simulink model "Cyber_Physical_Microgrid"  (R2024b)
settings: Solver=VariableStepAuto  StartTime=0.0  StopTime=270  RelTol=1e-3
values from neighbouring files (symbols this model uses):
  Bat =     [initData.mat]
  droopFC1 = 0.05    [initData.mat]
  droopFC2 = 0.05    [initData.mat]
  droopP2 = 0.05    [initData.mat]
  droopQ1 = 0.05    [initData.mat]
  droopQ2 = 0.05    [initData.mat]
  Pref2 = 0.8    [initData.mat]
  Qref1 = 0    [initData.mat]
  Qref2 = 0    [initData.mat]
  timeACLoadCurtail = 200    [initData.mat]
  timeSolarCurtail = 200    [initData.mat]
  Ts = 5e-05    [initData.mat]
  Ts_AC = 0.0002    [initData.mat]
  Ts_DC = 0.001    [initData.mat]
  volt2 = [270.467186401 250.166401688 246.278575679 243.847178474 242.073246789 240.654489675 239.457734124 238.414696845 237.485238449 236.643553985 235.871256975 235.151075236 ... (161 elements, 1x161)]    [initData.mat]
undefined symbols (not defined in the file or in its folder): BattTempBp, CapLUTBp, CapSOCBp, DiscIntNeverNeededParam, Em, Np, Ns, RInt, Tc_Batt
libraries: nesl_utility x55, fl_lib x52, ee_lib x39, modbuslib x16, spsRMSLib x8, simulink x5, spsFourierLib x2, batteryecm_lib x1, eeTransforms x1
(part 1 of 3)
settings Model: Creator=dines  LastModifiedBy=dines
settings ConfigSetCC: ModbusTableInfo=[]

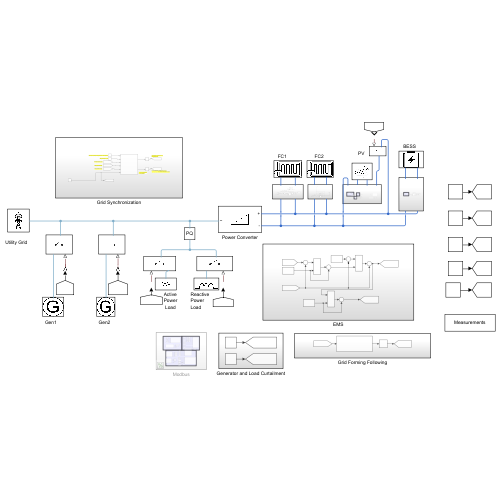
[thumbnail: Simulink's stored preview of the top-level diagram]
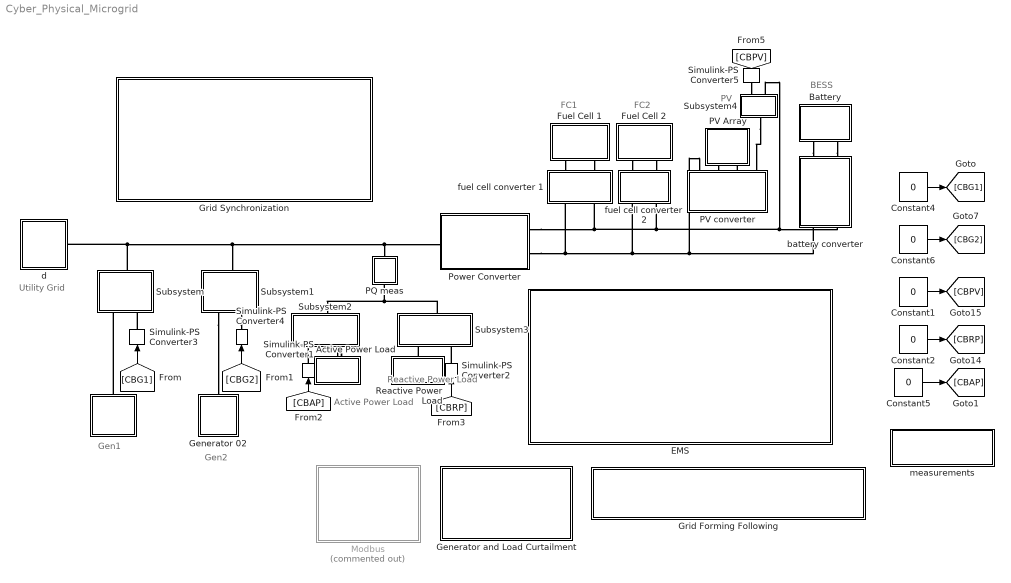
== system Cyber_Physical_Microgrid ==
  note: Gen1
  note: BESS
  note: PV
  note: FC1
  note: Reactive
      | Power
      | Load
  note: Gen2
  note: Active
      | Power
      |  Load
  note: FC2
  note: Utility Grid
  " " : Subsystem
      mask Display: image('generator.jpeg');
  Active Power Load : Subsystem
      mask Display: image('Resistor_symbol_America.svg.png');
  Battery : Subsystem
      mask Display: image('46518.png');
  Constant{1..2,4..6} (5 alike) : Constant  Value=0
  EMS : Subsystem
  Fuel Cell 1 : Subsystem
      mask Display: image('6255645.png');
  Fuel Cell 2 : Subsystem
      mask Display: image('6255645.png');
  Generator 02 : Subsystem
      mask Display: image('generator.jpeg');
  Generator and Load Curtailment : Subsystem
  Grid Forming Following : Subsystem
  Grid Synchronization : Subsystem
  Modbus : Subsystem  Commented=on
  PQ meas : Subsystem
      mask Display: disp('PQ')
  PV Array : Subsystem
      mask Display: image('solar-panel-icon-design-renewable-energy-sign-and-symbol-vector.jpg');
  PV converter : Subsystem
  Power Converter : Subsystem
      mask Display: image('743.s.png');
  Reactive Power Load : Subsystem
      mask Display: image('Inductor_symbol.svg.png');
  Simulink-PS Converter{1..5} (5 alike) : nesl_utility/Simulink-PS Converter  PhysicalDomain=network_engine_domain  SubClassName=ps_input  LeftPortType=input  RightPortType=output  PseudoPeriodic=off  Frequencies=[]  NoiseDistribution=none  NoiseParameters=[]  Unit=1  AffineConversion=off  FilteringAndDerivatives=provide  SimscapeFilterOrder=1  InputFilterTimeConstant=0.001  UdotUserProvided=0
  Subsystem : Subsystem
      mask Display: image('p0dz3vs9.png');
  Subsystem1 : Subsystem
      mask Display: image('p0dz3vs9.png');
  Subsystem2 : Subsystem
      mask Display: image('p0dz3vs9.png');
  Subsystem3 : Subsystem
      mask Display: image('p0dz3vs9.png');
  Subsystem4 : Subsystem
      mask Display: image('p0dz3vs9.png');
  battery converter : Subsystem
  d : Subsystem
      mask Display: image('utility.jpg');
  fuel cell converter 1 : Subsystem
  fuel cell converter 2 : Subsystem
  measurements : Subsystem
      mask Display: disp('Measurements')
  wires:
  [CBG2] -> Simulink-PS Converter4/1
  [CBG1] -> Simulink-PS Converter3/1
  Constant6/1 -> [CBG2]
  [CBAP] -> Simulink-PS Converter1/1
  Constant2/1 -> [CBRP]
  Constant1/1 -> [CBPV]
  [CBRP] -> Simulink-PS Converter2/1
  Constant4/1 -> [CBG1]
  Constant5/1 -> [CBAP]
  connections:
  fuel cell converter 2/RConn2 -- Subsystem4/LConn2 -- battery converter/RConn2 -- fuel cell converter 1/RConn2 -- Power Converter/RConn1
  PQ meas/LConn1 -- Power Converter/LConn1 -- Subsystem/RConn1 -- d/RConn1 -- Subsystem1/RConn1
  PV converter/LConn1 -- Power Converter/RConn2 -- fuel cell converter 1/RConn1 -- fuel cell converter 2/RConn1 -- battery converter/RConn1
  PQ meas/RConn1 -- Subsystem2/RConn1 -- Subsystem3/RConn1
  Battery/RConn2 -- battery converter/LConn2
  Simulink-PS Converter5/RConn1 -- Subsystem4/LConn1
  Simulink-PS Converter3/RConn1 -- Subsystem/LConn2
  Simulink-PS Converter1/RConn1 -- Subsystem2/LConn1
  PV converter/LConn3 -- PV Array/LConn2
  PV Array/LConn1 -- PV converter/LConn2
  Reactive Power Load/LConn1 -- Subsystem3/LConn1
  " "/RConn1 -- Subsystem/LConn1
  Subsystem2/LConn2 -- Active Power Load/LConn1
  Subsystem1/LConn2 -- Simulink-PS Converter4/RConn1
  Fuel Cell 1/RConn2 -- fuel cell converter 1/LConn2
  Battery/RConn1 -- battery converter/LConn1
  Fuel Cell 1/RConn1 -- fuel cell converter 1/LConn1
  Fuel Cell 2/RConn1 -- fuel cell converter 2/LConn1
  Fuel Cell 2/RConn2 -- fuel cell converter 2/LConn2
  Simulink-PS Converter2/RConn1 -- Subsystem3/LConn2
  Subsystem1/LConn1 -- Generator 02/RConn1
  Subsystem4/RConn1 -- PV converter/LConn4

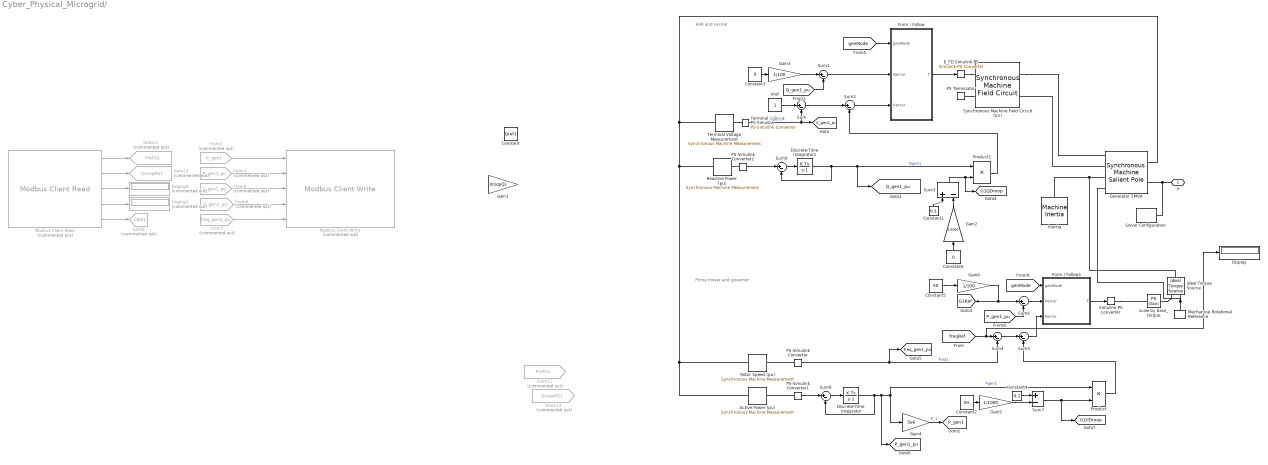
== system Cyber_Physical_Microgrid/  ==
  note: Prime mover
      | and governor
  note: AVR and exciter
  "Active Power (pu) " : ee_lib/Electromechanical/Synchronous/Synchronous Machine Measurement  output_idx=12
      settings: InternalSimscapePortConfiguration="{\"Bottom\":[],\"Left\":[{\"id\":\"pu_input\",\"label\":\"pu\",\"type\":\"input\"}],\"Right\":[{\"id\":\"pu_output\",\"label\":\"o\",\"type\":\"output\"}],\"Top\":[]}"
  Constant : Constant  Value=Qref1
  Constant1 : Constant  Value=0.1
  Constant2 : Constant  Value=50
  Constant3 : Constant  Value=0
  Constant4 : Constant  Value=0.1
  Constant5 : Constant  Value=50
  Constant6 : Constant  Value=0
  Discrete-Time Integrator : DiscreteIntegrator  gainval=20  SampleTime=Ts_AC  ICPrevOutput=DiscIntNeverNeededParam  ICPrevScaledInput=DiscIntNeverNeededParam
  Discrete-Time Integrator1 : DiscreteIntegrator  gainval=20  SampleTime=Ts_AC  ICPrevOutput=DiscIntNeverNeededParam  ICPrevScaledInput=DiscIntNeverNeededParam
  Display : Display
  Display2 : Display  Commented=on
      settings: Format=decimal (Stored Integer)  Decimation=4
  Display6 : Display  Commented=on
      settings: Format=decimal (Stored Integer)  Decimation=4
  "E_FD Simulink-PS " : nesl_utility/Simulink-PS Converter  PhysicalDomain=network_engine_domain  SubClassName=ps_input  LeftPortType=input  RightPortType=output  PseudoPeriodic=off  Frequencies=[]  NoiseDistribution=none  NoiseParameters=[]  Unit=1  AffineConversion=off  FilteringAndDerivatives=provide  SimscapeFilterOrder=1  InputFilterTimeConstant=.001  UdotUserProvided=0
  Form / Follow : Subsystem
  Form / Follow1 : Subsystem
  From11 : From  Commented=on  GotoTag=PrefG1
  From12 : From  Commented=on  GotoTag=DroopPG1
  From2 : From  Commented=on  GotoTag=P_gen1  TagVisibility=global
  From3 : From  Commented=on  GotoTag=P_gen1_pu  TagVisibility=global
  From4 : From  Commented=on  GotoTag=V_gen1_pu  TagVisibility=global
  From6 : From  Commented=on  GotoTag=Q_gen1_pu  TagVisibility=global
  From7 : From  Commented=on  GotoTag=freq_gen1_pu  TagVisibility=global
  Gain1 : Gain  Gain=droopQ1
  Gain2 : Gain  Gain=1/1000
  Gain3 : Gain  Gain=1/100
  Gain4 : Gain  Gain=5e6
  Gain5 : Gain  Gain=1/1000
  Gain6 : Gain  Gain=1/100
  Generator 5MVA : ee_lib/Electromechanical/Synchronous/Synchronous Machine Salient Pole  port_option=ee.enum.threePhasePort.composite  SRated=5e6 A*V  VRated=6600 V  FRated=50 Hz  nPolePairs=4  param_option=ee.enum.sm.parameterization.standard  fieldCircuitParameterization_option=ee.enum.sm.fieldparameterization.current  baseEfd=216.54 V  baseIfd=50 A  zero_sequence=ee.enum.park.zerosequence.exclude  axes_param=ee.enum.rotorangle.daxis  Ladu=0.9  Laqu=0.55  L0=0.15  Ll=0.15  Ra=0.011  Lfd=0.2571  Rfd=0.0006  L1d=0.2  R1d=0.0354  L1q=0.2567  R1q=0.0428  Xl=0.15  Xd=1.05  Xq=0.7  X0=0.15  Xdd=0.35  Xddd=0.25  Xqdd=0.325  d_option=ee.enum.circuit.open  Td0d=5.25 s  Tdd=1.75 s  Td0dd=0.03 s  Tddd=0.0214 s  q_option=ee.enum.circuit.open  Tq0dd=0.05 s  Tqdd=0.0232 s  saturation_option=ee.enum.saturation.exclude  saturation_ifd=[0.00, 0.48, 0.76, 1.38, 1.79]  saturation_Vag=[0.00, 0.43, 0.59, 0.71, 0.76]  initialization_option=ee.enum.sm.initialization.electrical  source_type=ee.enum.sm.load_flow_source_type.Swing  Vmag0=6600 V  Vang0=0 deg  Pt0=0.5 A*V  Qt0=0 A*V  minimum_pu=0.95  phase_search_range=[-inf, inf] deg  gmin=1e-6 S  connection_option=ee.enum.Connection.wye  num_q_dampers=1  rotor_offset=-pi / 2 rad  pu_psid_specify=on  pu_psid_priority=High  pu_psid=0  pu_psid_nominal_specify=off  pu_psid_nominal_value=1  pu_psid_nominal_unit=1  pu_psiq_specify=on  pu_psiq_priority=High  pu_psiq=0  pu_psiq_nominal_specify=off  pu_psiq_nominal_value=1  pu_psiq_nominal_unit=1  pu_psifd_specify=on  pu_psifd_priority=High  pu_psifd=0  pu_psifd_nominal_specify=off  pu_psifd_nominal_value=1  pu_psifd_nominal_unit=1  pu_psi1d_specify=on  pu_psi1d_priority=High  pu_psi1d=0  pu_psi1d_nominal_specify=off  pu_psi1d_nominal_value=1  pu_psi1d_nominal_unit=1  pu_psi1q_specify=on  pu_psi1q_priority=High  pu_psi1q=0  pu_psi1q_nominal_specify=off  pu_psi1q_nominal_value=1  pu_psi1q_nominal_unit=1  angular_position_diff_specify=on  angular_position_diff_priority=High  angular_position_diff=0 deg  angular_position_diff_nominal_specify=off  angular_position_diff_nominal_value=1  angular_position_diff_nominal_unit=deg  Tmeas=298.15 K  alpha=3.93e-3 1/K  stator_thermal_mass=100 J/K  rotor_thermal_mass=200 J/K  temperatureA_specify=off  temperatureA_priority=High  temperatureA=25 degC  temperatureA_nominal_specify=off  temperatureA_nominal_value=1  temperatureA_nominal_unit=degC  temperatureB_specify=off  temperatureB_priority=High  temperatureB=25 degC  temperatureB_nominal_specify=off  temperatureB_nominal_value=1  temperatureB_nominal_unit=degC  temperatureC_specify=off  temperatureC_priority=High  temperatureC=25 degC  temperatureC_nominal_specify=off  temperatureC_nominal_value=1  temperatureC_nominal_unit=degC  temperatureR_specify=off  temperatureR_priority=High  temperatureR=25 degC  temperatureR_nominal_specify=off  temperatureR_nominal_value=1  temperatureR_nominal_unit=degC
      settings: LogSimulationData=on  InternalSimscapePortConfiguration="{\"Bottom\":[],\"Left\":[{\"id\":\"fd_p\",\"label\":\"fd+\",\"type\":\"foundation.electrical.electrical\"},{\"id\":\"fd_n\",\"label\":\"fd-\",\"type\":\"foundation.electrical.electrical\"},{\"id\":\"R\",\"label\":\"R\",\"type\":\"foundation.mechanical.rotational.rotational\"},{\"id\":\"C\",\"label\":\"C\",\"type\":\"foundation.mechanical.rotational.rotational\"}],\"Right\":[{\"id\":\"pu_output\",\"label\":\"pu\",\"type\":\"output\"},{\"id\":\"N\",\"label\":\"~\",\"type\":\"foundation.electrical.three_phase\"}],\"Top\":[]}"
  Goto12 : Goto  Commented=on  GotoTag=PrefG1  TagVisibility=global
  Goto13 : Goto  Commented=on  GotoTag=DroopPG1  TagVisibility=global
  Goto8 : Goto  Commented=on  GotoTag=CBG1  TagVisibility=global
  Ideal Torque Source : fl_lib/Mechanical/Mechanical Sources/Ideal Torque Source
  Inertia : ee_lib/Electromechanical/Mechanical/Machine Inertia  SRated=5e6 V*A  FRated=50 Hz  nPolePairs=4  inertia_option=2  J=27548 kg*m^2  H=3.525 s*W/V/A  damper_option=2  D=39.0509 N*m/(rad/s)  pu_D=0.01  initialization_option=2  fMechanical0=50 Hz  fElectrical0=50 Hz
      settings: LogSimulationData=on  InternalSimscapePortConfiguration="{\"Bottom\":[],\"Left\":[{\"id\":\"R\",\"label\":\"R\",\"type\":\"foundation.mechanical.rotational.rotational\"}],\"Right\":[],\"Top\":[]}"
  Mechanical Rotational Reference : fl_lib/Mechanical/Rotational Elements/Mechanical Rotational Reference
  Modbus Client Read : modbuslib/Modbus Client Read  Commented=on  RetainClient=No Modbus client available  ClientList=No Modbus client available  ConnectionEndpoint=No Modbus client selected  ServerId=1  RegisterTable={ '1', 'PrefG1', '21', 'Holding Register', 'double', '1'; '2', 'DroopPG1', '25', 'Holding Register', 'double', '1'; '3', 'QrefG1', '29', 'Holding Register', 'double', '1'; '4', 'DroopQG1', '34', 'Holding Register', 'double', '1'; '5', 'CBG1', '38', 'Coil', 'bit', '1' }  SampleTime=1
  Modbus Client Write : modbuslib/Modbus Client Write  Commented=on  RetainClient=No Modbus client available  ClientList=No Modbus client available  ConnectionEndpoint=No Modbus client selected  ServerId=1  RegisterTable={ '1', 'P_gen1', '1', 'Holding Register', 'double'; '2', 'P_gen1_pu', '5', 'Holding Register', 'double'; '3', 'V_gen1_pu', '9', 'Holding Register', 'double'; '4', 'Q_gen1_pu', '13', 'Holding Register', 'double'; '5', 'freq_gen1_pu', '17', 'Holding Register', 'double' }  SampleTime=1
  PS Terminator : fl_lib/Physical Signals/Sinks/PS Terminator
  PS-Simulink Converter : nesl_utility/PS-Simulink Converter  PhysicalDomain=network_engine_domain  SubClassName=ps_output  LeftPortType=input  RightPortType=output  PseudoPeriodic=off  Frequencies=[]  VectorFormat=1-D array  Unit=inherit  AffineConversion=off
  PS-Simulink Converter1 : nesl_utility/PS-Simulink Converter  PhysicalDomain=network_engine_domain  SubClassName=ps_output  LeftPortType=input  RightPortType=output  PseudoPeriodic=off  Frequencies=[]  VectorFormat=1-D array  Unit=inherit  AffineConversion=off
  PS-Simulink Converter2 : nesl_utility/PS-Simulink Converter  PhysicalDomain=network_engine_domain  SubClassName=ps_output  LeftPortType=input  RightPortType=output  PseudoPeriodic=off  Frequencies=[]  VectorFormat=1-D array  Unit=inherit  AffineConversion=off
  Product : Product
  Product1 : Product
  Reactive Power (pu) : ee_lib/Electromechanical/Synchronous/Synchronous Machine Measurement  output_idx=13
      settings: InternalSimscapePortConfiguration="{\"Bottom\":[],\"Left\":[{\"id\":\"pu_input\",\"label\":\"pu\",\"type\":\"input\"}],\"Right\":[{\"id\":\"pu_output\",\"label\":\"o\",\"type\":\"output\"}],\"Top\":[]}"
  Rotor Speed (pu) : ee_lib/Electromechanical/Synchronous/Synchronous Machine Measurement  output_idx=4
      settings: InternalSimscapePortConfiguration="{\"Bottom\":[],\"Left\":[{\"id\":\"pu_input\",\"label\":\"pu\",\"type\":\"input\"}],\"Right\":[{\"id\":\"pu_output\",\"label\":\"o\",\"type\":\"output\"}],\"Top\":[]}"
  Simulink-PS Converter : nesl_utility/Simulink-PS Converter  PhysicalDomain=network_engine_domain  SubClassName=ps_input  LeftPortType=input  RightPortType=output  PseudoPeriodic=off  Frequencies=[]  NoiseDistribution=none  NoiseParameters=[]  Unit=1  AffineConversion=off  FilteringAndDerivatives=provide  SimscapeFilterOrder=1  InputFilterTimeConstant=0.001  UdotUserProvided=0
  Solver Configuration : nesl_utility/Solver Configuration  PhysicalDomain=network_engine_domain  SubClassName=solver  LeftPortType=input  RightPortType=generic  Tones=[]  Harmonics=[]  SimulateNoise=off  Profile=off  UseLocalSampling=off  EnableSwitchedLinearOptims=on  FrequencyDomain=off  UseCCode=off  RelTol=0.001  AbsTol=1e-06  MinStep=1e-09  ToWorkspace=off  RevertToSquareIcSolve=off  NumHomotopyIterations=100  PhasorMode=off  PhasorModeNumHarmonics=1  ConsistencySolver=NEWTON_FTOL  IndexReductionMethod=DerivativeReplacement  DoDC=off  ResidualTolerance=1e-09  ConsistencyTolSource=GLOBAL  ConsistencyAbsTol=0.001  ConsistencyRelTol=0.001  ConsistencyTolFactor=0.001  UseLocalSolver=on  LocalSolverChoice=NE_PARTITIONING_ADVANCER  ResolveIndetEquations=on  FunctionEvalNumThread=1  LocalSolverSampleTime=Ts_DC  DoFixedCost=on  MaxNonlinIter=1  MaxModeIter=2  ComputeImpulses=off  ImpulseIterations=2  LinearAlgebra=auto  LinearAlgebraNumThread=0  EquationFormulation=NE_TIME_EF  DelaysMemoryBudget=1024  AutomaticFiltering=on  FilteringTimeConstant=0.001  PartitionStorageMethod=AS_NEEDED  PartitionMemoryBudget=1024  PartitionMethod=ROBUST  MultibodyUseLocalSolver=off  MultibodyLocalSolverChoice=ODE1  MultibodyLocalSolverSampleTime=0.001
  Sum{,1..2,4..6,8..9} (8 alike) : Sum  Inputs=|+-
  Sum3 : Sum  Inputs=+-
  Sum7 : Sum  Inputs=+-
  Synchronous Machine Field Circuit (pu) : ee_lib/Electromechanical/Synchronous/Synchronous Machine Field Circuit  unit_option=ee.enum.unit.pu  SRated=5e6 V*A  FRated=50 Hz  fieldCircuitParameterization_option=2  baseEfd=92.95 V  baseIfd=50 A  parameterization_option=2  Ladu=1.66  Rfd=0.0006  Xl=0.15  Xd=1.05  Xdd=0.35  Xddd=0.23  d_option=ee.enum.circuit.open  Td0d=5.25 s  Tdd=1.3260 s  Td0dd=0.03 s  Tddd=0.0230 s
      settings: LogSimulationData=on  InternalSimscapePortConfiguration="{\"Bottom\":[],\"Left\":[{\"id\":\"Efd_pu\",\"label\":\"Efd_pu\",\"type\":\"input\"},{\"id\":\"Ifd_pu\",\"label\":\"Ifd_pu\",\"type\":\"output\"}],\"Right\":[{\"id\":\"fd_p\",\"label\":\"fd+\",\"type\":\"foundation.electrical.electrical\"},{\"id\":\"fd_n\",\"label\":\"fd-\",\"type\":\"foundation.electrical.electrical\"}],\"Top\":[]}"
  Terminal Voltage Measurement : ee_lib/Electromechanical/Synchronous/Synchronous Machine Measurement  output_idx=14
      settings: LogSimulationData=on  InternalSimscapePortConfiguration="{\"Bottom\":[],\"Left\":[{\"id\":\"pu_input\",\"label\":\"pu\",\"type\":\"input\"}],\"Right\":[{\"id\":\"pu_output\",\"label\":\"o\",\"type\":\"output\"}],\"Top\":[]}"
  Terminal Voltage PS-Simulink : nesl_utility/PS-Simulink Converter  PhysicalDomain=network_engine_domain  SubClassName=ps_output  LeftPortType=input  RightPortType=output  PseudoPeriodic=off  Frequencies=[]  VectorFormat=1-D array  Unit=1  AffineConversion=off
  Vref : Constant  SampleTime=Ts_AC
  scale by base_torque : fl_lib/Physical Signals/Functions/PS Gain  gain=63661.97724 N*m
  a : PMIOPort  Side=Right
  tag scope: G1PDroop=global, G1QDroop=global, G1Ref=global, P_gen1=global, P_gen1_pu=global, Q_gen1_pu=global, V_gen1_pu=global, freq_gen1_pu=global
  wires:
  Product1/1 -> Sum2/2
  Gain3/1 -> Sum1/1
  Gain2/1 -> Sum3/2
  Sum3/1 -> [G1QDroop], Product1/2
  Constant1/1 -> Sum3/1
  Constant6/1 -> Gain2/1
  Form / Follow/1(T) -> "E_FD Simulink-PS "/1
  [Q_gen1_pu] -> Sum1/2
  [genMode] -> Form / Follow/1(genMode)
  Sum1/1 -> Form / Follow/2(Qerror)
  Discrete-Time Integrator1/1 -> Product1/1, [Q_gen1_pu], Sum9/2  "Qgen1"
  Terminal Voltage PS-Simulink/1 -> [V_gen1_pu], Sum/2  "Vgen1"
  Sum2/1 -> Form / Follow/3(Verror)
  Sum/1 -> Sum2/1
  Vref/1 -> Sum/1
  Modbus Client Read/1 -> Goto12/1
  From7/1 -> Modbus Client Write/5
  From6/1 -> Modbus Client Write/4
  From4/1 -> Modbus Client Write/3
  From3/1 -> Modbus Client Write/2
  From2/1 -> Modbus Client Write/1
  Gain6/1 -> Sum6/1, [G1Ref]
  Sum7/1 -> [G1PDroop], Product/2
  Gain5/1 -> Sum7/2
  Constant4/1 -> Sum7/1
  Form / Follow1/1(T) -> Simulink-PS Converter/1
  [genMode] -> Form / Follow1/1(genMode)
  Sum6/1 -> Form / Follow1/2(Perror)
  Sum5/1 -> Form / Follow1/3(Ferror)
  [P_gen1_pu] -> Sum6/2
  Gain4/1 -> [P_gen1]  "P_1"
  Discrete-Time Integrator/1 -> Gain4/1, Product/1, [P_gen1_pu], Sum8/2  "Pgen1"
  Product/1 -> Sum5/2
  Sum4/1 -> Sum5/1
  [freqRef] -> Display/1, Sum4/1
  PS-Simulink Converter/1 -> [freq_gen1_pu], Sum4/2  "freq1"
  Modbus Client Read/2 -> Goto13/1
  Modbus Client Read/5 -> Goto8/1
  Modbus Client Read/3 -> Display6/1
  Modbus Client Read/4 -> Display2/1
  Constant2/1 -> Gain5/1
  Constant5/1 -> Gain6/1
  PS-Simulink Converter1/1 -> Sum8/1
  Sum8/1 -> Discrete-Time Integrator/1
  Constant3/1 -> Gain3/1
  PS-Simulink Converter2/1 -> Sum9/1
  Sum9/1 -> Discrete-Time Integrator1/1
  connections:
  Synchronous Machine Field Circuit (pu)/RConn1 -- Generator 5MVA/LConn1
  Ideal Torque Source/LConn1 -- Generator 5MVA/LConn3 -- Inertia/LConn1
  Mechanical Rotational Reference/LConn1 -- Ideal Torque Source/RConn2 -- Generator 5MVA/LConn4
  Solver Configuration/RConn1 -- a/RConn1 -- Generator 5MVA/RConn2
  PS-Simulink Converter2/LConn1 -- Reactive Power (pu)/RConn1
  Terminal Voltage Measurement/RConn1 -- Terminal Voltage PS-Simulink/LConn1
  Rotor Speed (pu)/LConn1 -- "Active Power (pu) "/LConn1 -- Generator 5MVA/RConn1 -- Terminal Voltage Measurement/LConn1 -- Reactive Power (pu)/LConn1
  "E_FD Simulink-PS "/RConn1 -- Synchronous Machine Field Circuit (pu)/LConn1
  PS Terminator/LConn1 -- Synchronous Machine Field Circuit (pu)/LConn2
  Generator 5MVA/LConn2 -- Synchronous Machine Field Circuit (pu)/RConn2
  PS-Simulink Converter1/LConn1 -- "Active Power (pu) "/RConn1
  PS-Simulink Converter/LConn1 -- Rotor Speed (pu)/RConn1
  scale by base_torque/RConn1 -- Ideal Torque Source/RConn1
  Simulink-PS Converter/RConn1 -- scale by base_torque/LConn1

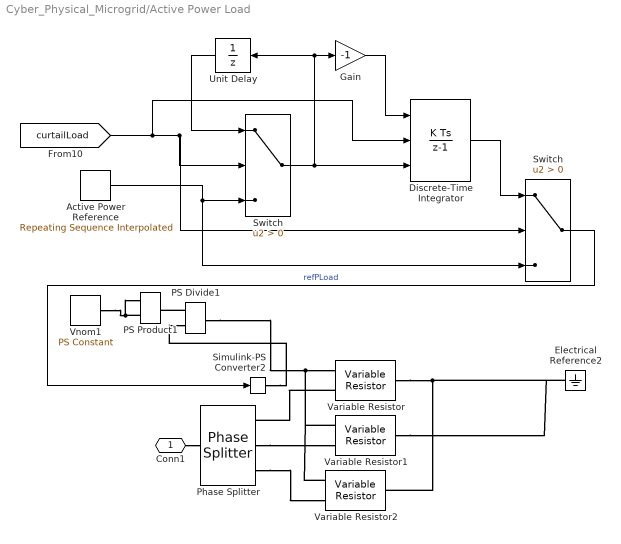
== system Cyber_Physical_Microgrid/Active Power Load ==
  Active Power Reference : simulink/Sources/Repeating Sequence Interpolated  OutValues=[1 1 10e6 10e6]  TimeValues=[0 1 5 500]  LookUpMeth=Interpolation-Use End Values  tsamp=Ts_AC  OutMin=[]  OutMax=[]  OutDataTypeStr=double  OutputDataTypeScalingMode=double  OutDataType=fixdt(0,8)  OutScaling=2^-10
  Discrete-Time Integrator : DiscreteIntegrator  gainval=1e-2  ExternalReset=rising  InitialConditionSource=external  SampleTime=-1  LimitOutput=on  LowerSaturationLimit=6e6  ICPrevOutput=DiscIntNeverNeededParam  ICPrevScaledInput=DiscIntNeverNeededParam
  Electrical Reference2 : fl_lib/Electrical/Electrical Elements/Electrical Reference
  Gain : Gain  Gain=-1
  PS Divide1 : fl_lib/Physical Signals/Functions/PS Divide
  PS Product1 : fl_lib/Physical Signals/Functions/PS Product
  Phase Splitter : ee_lib/Connectors & References/Phase Splitter
  Simulink-PS Converter2 : nesl_utility/Simulink-PS Converter  PhysicalDomain=network_engine_domain  SubClassName=ps_input  LeftPortType=input  RightPortType=output  PseudoPeriodic=off  Frequencies=[]  NoiseDistribution=none  NoiseParameters=[]  Unit=W  AffineConversion=off  FilteringAndDerivatives=provide  SimscapeFilterOrder=1  InputFilterTimeConstant=0.001  UdotUserProvided=0
  Switch : Switch  Criteria=u2 > Threshold  SaturateOnIntegerOverflow=off  InputSameDT=off
  "Switch " : Switch  Criteria=u2 > Threshold  SaturateOnIntegerOverflow=off  InputSameDT=off
  Unit Delay : UnitDelay  SampleTime=-1  HasFrameUpgradeWarning=on
  Variable Resistor : fl_lib/Electrical/Electrical Elements/Variable Resistor  Rmin=0 Ohm  thermalEnable=false  thermal_mass=1 J/K  i_specify=off  i_priority=None  i=0 A  i_nominal_specify=off  i_nominal_value=1  i_nominal_unit=A  v_specify=off  v_priority=None  v=0 V  v_nominal_specify=off  v_nominal_value=1  v_nominal_unit=V  T_specify=off  T_priority=None  T=300 K  T_nominal_specify=off  T_nominal_value=1  T_nominal_unit=K
  Variable Resistor1 : fl_lib/Electrical/Electrical Elements/Variable Resistor  Rmin=0 Ohm  thermalEnable=false  thermal_mass=1 J/K  i_specify=off  i_priority=None  i=0 A  i_nominal_specify=off  i_nominal_value=1  i_nominal_unit=A  v_specify=off  v_priority=None  v=0 V  v_nominal_specify=off  v_nominal_value=1  v_nominal_unit=V  T_specify=off  T_priority=None  T=300 K  T_nominal_specify=off  T_nominal_value=1  T_nominal_unit=K
  Variable Resistor2 : fl_lib/Electrical/Electrical Elements/Variable Resistor  Rmin=0 Ohm  thermalEnable=false  thermal_mass=1 J/K  i_specify=off  i_priority=None  i=0 A  i_nominal_specify=off  i_nominal_value=1  i_nominal_unit=A  v_specify=off  v_priority=None  v=0 V  v_nominal_specify=off  v_nominal_value=1  v_nominal_unit=V  T_specify=off  T_priority=None  T=300 K  T_nominal_specify=off  T_nominal_value=1  T_nominal_unit=K
  Vnom1 : fl_lib/Physical Signals/Sources/PS Constant  constant=6600 V
  Conn1 : PMIOPort  Side=Left
  wires:
  "Switch "/1 -> Simulink-PS Converter2/1  "refPLoad"
  Gain/1 -> Discrete-Time Integrator/1
  Active Power Reference/1 -> "Switch "/3, Switch/3
  Unit Delay/1 -> Switch/1
  Switch/1 -> Unit Delay/1, Gain/1, Discrete-Time Integrator/3
  [curtailLoad] -> "Switch "/2, Switch/2, Discrete-Time Integrator/2
  Discrete-Time Integrator/1 -> "Switch "/1
  connections:
  Conn1/RConn1 -- Phase Splitter/LConn1
  PS Product1/LConn2 -- Vnom1/RConn1 -- PS Product1/LConn1
  Phase Splitter/RConn2 -- Variable Resistor1/LConn2
  Simulink-PS Converter2/RConn1 -- PS Divide1/LConn2
  Variable Resistor/RConn1 -- Electrical Reference2/LConn1 -- Variable Resistor1/RConn1 -- Variable Resistor2/RConn1
  PS Divide1/RConn1 -- Variable Resistor2/LConn1 -- Variable Resistor1/LConn1 -- Variable Resistor/LConn1
  Variable Resistor/LConn2 -- Phase Splitter/RConn1
  PS Divide1/LConn1 -- PS Product1/RConn1
  Phase Splitter/RConn3 -- Variable Resistor2/LConn2

== system Cyber_Physical_Microgrid/Battery ==
  Battery1 : batteryecm_lib/Battery (Table-Based)  SOC_vec=Bat.CapSOCBp  T_dependence=simscape.enum.tablebattery.temperature_dependence.yes  prm_dir=simscape.enum.tablebattery.prm_dir.noCurrentDirectionality  T_vec=Bat.BattTempBp K  V0_mat=Bat.noLoadV*18.32 V  V0_vec=Ns*interp1(CapLUTBp,Em,CapSOCBp) V  V_range=[0, inf] V  R0_mat=Bat.R0 Ohm  R0_vec=RInt*Ns/Np Ohm  R0_dis_mat=[.03, .015, .002; .04, .017, .008; .039, .012, .006; .027, .013, .021] Ohm  R0_dis_vec=[.015, .017, .012, .013] Ohm  R0_ch_mat=[.03, .015, .002; .04, .017, .008; .039, .012, .006; .027, .013, .021] Ohm  R0_ch_vec=[.015, .017, .012, .013] Ohm  AH=Bat.AH A*hr  prm_leak=simscape.enum.tablebattery.prm_leak.disabled  Rleak_vec=[8000, 7000, 6000] Ohm  Rleak=7e3 Ohm  extrapolation_option=simscape.enum.extrapolation.linear  SOC_port=simscape.enum.tablebattery.enable.yes  prm_dyn=simscape.enum.tablebattery.prm_dyn.off  R1_mat=(RInt').*Ns/Np Ohm  R1_vec=[.076, .022, .007, .043] Ohm  tau1_mat=Tc_Batt*ones(1,length(CapSOCBp))'*ones(1,length(BattTempBp)) s  tau1_vec=[148, 110, 27, 22] s  R2_mat=[.014, .382, .407; .028, .006, .007; .014, .007, .006; .333, .956, .912] Ohm  R2_vec=[.382, .006, .007, .956] Ohm  tau2_mat=[1, 44, 5644; 11, 24, 506; 2, 14, 330; 3310, 13419, 30216] s  tau2_vec=[44, 24, 14, 13419] s  R3_mat=[.014, .382, .407; .028, .006, .007; .014, .007, .006; .333, .956, .912] Ohm  R3_vec=[.382, .006, .007, .956] Ohm  tau3_mat=[1, 44, 5644; 11, 24, 506; 2, 14, 330; 3310, 13419, 30216] s  tau3_vec=[44, 24, 14, 13419] s  R4_mat=[.014, .382, .407; .028, .006, .007; .014, .007, .006; .333, .956, .912] Ohm  R4_vec=[.382, .006, .007, .956] Ohm  tau4_mat=[1, 44, 5644; 11, 24, 506; 2, 14, 330; 3310, 13419, 30216] s  tau4_vec=[44, 24, 14, 13419] s  R5_mat=[.014, .382, .407; .028, .006, .007; .014, .007, .006; .333, .956, .912] Ohm  R5_vec=[.382, .006, .007, .956] Ohm  tau5_mat=[1, 44, 5644; 11, 24, 506; 2, 14, 330; 3310, 13419, 30216] s  tau5_vec=[44, 24, 14, 13419] s  prm_fade=simscape.enum.tablebattery.prm_fade.equations  N0=100  dV0=1e-3  dR0=1e-3  dAH=1e-3  dRleak=0  dR1=0  dR2=0  dR3=0  dR4=0  dR5=0  N0vec=[100, 200, 300]  Tfadevec=[298.15, 323.15] K  dV0vec=[0, 0, 0]  dR0vec=[0, 0, 0]  dAHvec=[0, 0, 0]  dRleakvec=[0, 0, 0]  dR1vec=[0, 0, 0]  dR2vec=[0, 0, 0]  dR3vec=[0, 0, 0]  dR4vec=[0, 0, 0]  dR5vec=[0, 0, 0]  dV0mat=[0, 0; 0, 0; 0, 0]  dR0mat=[0, 0; 0, 0; 0, 0]  dAHmat=[0, 0; 0, 0; 0, 0]  dRleakmat=[0, 0; 0, 0; 0, 0]  dR1mat=[0, 0; 0, 0; 0, 0]  dR2mat=[0, 0; 0, 0; 0, 0]  dR3mat=[0, 0; 0, 0; 0, 0]  dR4mat=[0, 0; 0, 0; 0, 0]  dR5mat=[0, 0; 0, 0; 0, 0]  prm_age_modeling=simscape.enum.tablebattery.prm_age_modeling.equation  storage_dt_age_vec=[0] d  storage_T_age_vec=[273] K  prm_age_OCV=simscape.enum.tablebattery.prm_age_OCV.OCV  OCV_age=0.9  SOC_age=0.6  prm_age_resistance=simscape.enum.tablebattery.prm_age.disabled  OCV_scaling_age_resistance=2.2134e6  OCV_offset_age_resistance=1.632e6  temp_exp_age_resistance=0.515833569 V  t_exp_age_resistance=0.75  T_age_vec_resistance=[273.15, 298.15, 323.15] K  dt_age_vec_resistance=[90, 180, 270, 360] d  dR0_age_vec=[0, 0, 0]  t_meas_dR0_age=100 d  dR0_age_mat=[0, 0, 0; 0, 0, 0; 0, 0, 0; 0, 0, 0]  prm_age_capacity=simscape.enum.tablebattery.prm_age.disabled  OCV_scaling_age_capacity=1.5097e07  OCV_offset_age_capacity=8.3625e06  temp_exp_age_capacity=0.6011 V  t_exp_age_capacity=0.75  T_age_vec_capacity=[273.15, 298.15, 323.15] K  dt_age_vec_capacity=[90, 180, 270, 360] d  dAH_age_vec=[0, 0, 0]  t_meas_dAH_age=100 d  dAH_age_mat=[0, 0, 0; 0, 0, 0; 0, 0, 0; 0, 0, 0]  thermal_port=simscape.enum.thermaleffects.omit  temperature=300 K  thermal_mass=30000 J/K  i_specify=off  i_priority=High  i=0 A  i_nominal_specify=off  i_nominal_value=1  i_nominal_unit=A  v_specify=off  v_priority=None  v=280 V  v_nominal_specify=off  v_nominal_value=1  v_nominal_unit=V  stateOfCharge_specify=on  stateOfCharge_priority=High  stateOfCharge=Bat.initSOC  stateOfCharge_nominal_specify=off  stateOfCharge_nominal_value=1  stateOfCharge_nominal_unit=1  num_cycles_specify=off  num_cycles_priority=High  num_cycles=0  num_cycles_nominal_specify=off  num_cycles_nominal_value=1  num_cycles_nominal_unit=1  cell_temperature_specify=off  cell_temperature_priority=High  cell_temperature=298.15 K  cell_temperature_nominal_specify=off  cell_temperature_nominal_value=1  cell_temperature_nominal_unit=K
      settings: InternalSimscapePortConfiguration="{\"Bottom\":[],\"Left\":[{\"id\":\"p\",\"label\":\"+\",\"type\":\"foundation.electrical.electrical\"},{\"id\":\"soc\",\"label\":\"SOC\",\"type\":\"output\"}],\"Right\":[{\"id\":\"n\",\"label\":\"-\",\"type\":\"foundation.electrical.electrical\"}],\"Top\":[]}"
  Current Sensor1 : fl_lib/Electrical/Electrical Sensors/Current Sensor
  Display : Display
  Display1 : Display
  Electrical Reference1 : fl_lib/Electrical/Electrical Elements/Electrical Reference
  PS-Simulink Converter : nesl_utility/PS-Simulink Converter  PhysicalDomain=network_engine_domain  SubClassName=ps_output  LeftPortType=input  RightPortType=output  PseudoPeriodic=off  Frequencies=[]  VectorFormat=1-D array  Unit=inherit  AffineConversion=off
  PS-Simulink Converter1 : nesl_utility/PS-Simulink Converter  PhysicalDomain=network_engine_domain  SubClassName=ps_output  LeftPortType=input  RightPortType=output  PseudoPeriodic=off  Frequencies=[]  VectorFormat=1-D array  Unit=inherit  AffineConversion=off
  PS-Simulink Converter4 : nesl_utility/PS-Simulink Converter  PhysicalDomain=network_engine_domain  SubClassName=ps_output  LeftPortType=input  RightPortType=output  PseudoPeriodic=off  Frequencies=[]  VectorFormat=1-D array  Unit=inherit  AffineConversion=off
  Resistor1 : fl_lib/Electrical/Electrical Elements/Resistor  R=1e-3 Ohm  i_specify=off  i_priority=None  i=0 A  i_nominal_specify=off  i_nominal_value=1  i_nominal_unit=A  v_specify=off  v_priority=None  v=0 V  v_nominal_specify=off  v_nominal_value=1  v_nominal_unit=V
  Terminator1 : Terminator
  Terminator2 : Terminator
  Voltage Sensor : fl_lib/Electrical/Electrical Sensors/Voltage Sensor
  Conn1 : PMIOPort  Side=Right
  Conn2 : PMIOPort  Port=2  Side=Right
  tag scope: SOC_batt=global
  wires:
  PS-Simulink Converter/1 -> [SOC_batt]  "SOC"
  PS-Simulink Converter4/1 -> Display1/1, Terminator2/1  "Ibatt_supply"
  PS-Simulink Converter1/1 -> Display/1, Terminator1/1  "Vbatt_supply"
  connections:
  Battery1/LConn1 -- Current Sensor1/LConn1
  PS-Simulink Converter4/LConn1 -- Current Sensor1/RConn1
  Conn1/RConn1 -- Resistor1/RConn1
  PS-Simulink Converter/LConn1 -- Battery1/LConn2
  Battery1/RConn1 -- Electrical Reference1/LConn1 -- Conn2/RConn1 -- Voltage Sensor/RConn2
  Voltage Sensor/LConn1 -- Resistor1/LConn1 -- Current Sensor1/RConn2
  PS-Simulink Converter1/LConn1 -- Voltage Sensor/RConn1

== system Cyber_Physical_Microgrid/EMS ==
  AC Load Limit (W) : Constant  Value=8e6  SampleTime=Ts_DC
  FC + PV limit (W) : Constant  Value=1.7e6  SampleTime=Ts_DC
  MinMax1 : MinMax  Function=max  Inputs=2
  MinMax2 : MinMax  Inputs=2
  MinMax3 : MinMax  Function=max  Inputs=2
  Power Transfer Limit (W) : Constant  Value=5e6  SampleTime=Ts_DC
  Sum{1..3,5} (4 alike) : Sum  Inputs=|+-
  Sum4 : Sum  Inputs=|++
  tag scope: P_AC_ref=global, P_batt_ref=global
  wires:
  Power Transfer Limit (W)/1 -> Sum2/1
  Sum1/1 -> MinMax1/1
  MinMax3/1 -> Sum3/1
  Sum5/1 -> MinMax2/2
  Sum4/1 -> MinMax3/1, [P_AC_ref]
  AC Load Limit (W)/1 -> Sum5/2, MinMax1/2
  [P_load] -> Sum1/1
  Sum2/1 -> MinMax2/1
  FC + PV limit (W)/1 -> Sum3/2, MinMax3/2
  MinMax2/1 -> Sum4/1
  MinMax1/1 -> Sum5/1
  [P_PV] -> Sum2/2, Sum4/2, Sum1/2
  Sum3/1 -> [P_batt_ref]

== system Cyber_Physical_Microgrid/Fuel Cell 1 ==
  Controlled Voltage Source : fl_lib/Electrical/Electrical Sources/Controlled Voltage Source
  Current Sensor : fl_lib/Electrical/Electrical Sensors/Current Sensor
  PS Lookup Table (1D) : fl_lib/Physical Signals/Lookup Tables/PS Lookup Table (1D)  x=curr A  f=volt2*20 V  interp_method=simscape.enum.interpolation.linear  extrap_method=simscape.enum.extrapolation.linear
  Resistor2 : fl_lib/Electrical/Electrical Elements/Resistor  R=1e-3 Ohm  i_specify=off  i_priority=None  i=0 A  i_nominal_specify=off  i_nominal_value=1  i_nominal_unit=A  v_specify=off  v_priority=None  v=0 V  v_nominal_specify=off  v_nominal_value=1  v_nominal_unit=V
  Conn1 : PMIOPort  Side=Right
  Conn2 : PMIOPort  Port=2  Side=Right
  connections:
  Controlled Voltage Source/RConn1 -- PS Lookup Table (1D)/RConn1
  Current Sensor/RConn2 -- Resistor2/LConn1
  Controlled Voltage Source/LConn1 -- Current Sensor/LConn1
  Current Sensor/RConn1 -- PS Lookup Table (1D)/LConn1
  Controlled Voltage Source/RConn2 -- Conn2/RConn1
  Conn1/RConn1 -- Resistor2/RConn1

== system Cyber_Physical_Microgrid/Fuel Cell 2 ==
  Controlled Voltage Source : fl_lib/Electrical/Electrical Sources/Controlled Voltage Source
  Current Sensor : fl_lib/Electrical/Electrical Sensors/Current Sensor
  PS Lookup Table (1D) : fl_lib/Physical Signals/Lookup Tables/PS Lookup Table (1D)  x=curr A  f=volt2*20 V  interp_method=simscape.enum.interpolation.linear  extrap_method=simscape.enum.extrapolation.linear
  Resistor2 : fl_lib/Electrical/Electrical Elements/Resistor  R=1e-3 Ohm  i_specify=off  i_priority=None  i=0 A  i_nominal_specify=off  i_nominal_value=1  i_nominal_unit=A  v_specify=off  v_priority=None  v=0 V  v_nominal_specify=off  v_nominal_value=1  v_nominal_unit=V
  Conn1 : PMIOPort  Side=Right
  Conn2 : PMIOPort  Port=2  Side=Right
  connections:
  Current Sensor/RConn2 -- Resistor2/LConn1
  Controlled Voltage Source/RConn1 -- PS Lookup Table (1D)/RConn1
  Current Sensor/RConn1 -- PS Lookup Table (1D)/LConn1
  Conn1/RConn1 -- Resistor2/RConn1
  Controlled Voltage Source/LConn1 -- Current Sensor/LConn1
  Controlled Voltage Source/RConn2 -- Conn2/RConn1

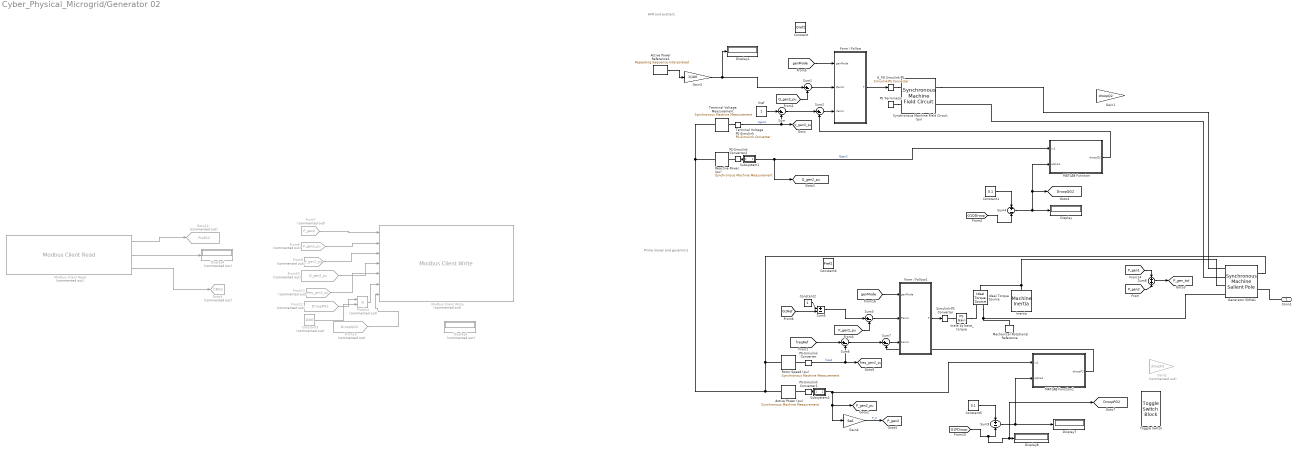
== system Cyber_Physical_Microgrid/Generator 02 ==
  note: Prime mover
      | and governor1
  note: AVR and exciter1
  "Active Power (pu) " : ee_lib/Electromechanical/Synchronous/Synchronous Machine Measurement  output_idx=12
      settings: InternalSimscapePortConfiguration="{\"Bottom\":[],\"Left\":[{\"id\":\"pu_input\",\"label\":\"pu\",\"type\":\"input\"}],\"Right\":[{\"id\":\"pu_output\",\"label\":\"o\",\"type\":\"output\"}],\"Top\":[]}"
  Active Power Reference1 : simulink/Sources/Repeating Sequence Interpolated  OutValues=[0 0 0 0 0 0]  TimeValues=[100 110 120 130 140 500]  LookUpMeth=Interpolation-Use End Values  tsamp=Ts_AC  OutMin=[]  OutMax=[]  OutDataTypeStr=double  OutputDataTypeScalingMode=double  OutDataType=fixdt(0,8)  OutScaling=2^-10
  Constant : Constant  Value=Qref2
  Constant1 : Constant  Value=0.1
  Constant2 : Constant
  Constant3 : Constant  Commented=on  Value=1000
  Constant4 : Constant  Value=Pref2
  Constant5 : Constant  Value=0.1
  Display{,1,7..8} (4 alike) : Display
  Display4 : Display  Commented=on
      settings: Format=decimal (Stored Integer)  Decimation=4
  Display9 : Display  Commented=on
  "E_FD Simulink-PS " : nesl_utility/Simulink-PS Converter  PhysicalDomain=network_engine_domain  SubClassName=ps_input  LeftPortType=input  RightPortType=output  PseudoPeriodic=off  Frequencies=[]  NoiseDistribution=none  NoiseParameters=[]  Unit=1  AffineConversion=off  FilteringAndDerivatives=provide  SimscapeFilterOrder=1  InputFilterTimeConstant=.001  UdotUserProvided=0
  Form / Follow : Subsystem
  Form / Follow1 : Subsystem
  From10 : From  Commented=on  GotoTag=Q_gen2_pu  TagVisibility=global
  From11 : From  Commented=on  GotoTag=freq_gen2_pu  TagVisibility=global
  From12 : From  Commented=on  GotoTag=DroopPG2  TagVisibility=global
  From13 : From  Commented=on  GotoTag=DroopQG2  TagVisibility=global
  From7 : From  Commented=on  GotoTag=P_gen2  TagVisibility=global
  From8 : From  Commented=on  GotoTag=P_gen2_pu  TagVisibility=global
  From9 : From  Commented=on  GotoTag=V_gen2_pu  TagVisibility=global
  Gain1 : Gain  Gain=droopQ2
  Gain2 : Gain  Commented=on  Gain=droopP2
  Gain3 : Gain  Gain=1/100
  Gain4 : Gain  Gain=5e6
  Generator 5MVA1 : ee_lib/Electromechanical/Synchronous/Synchronous Machine Salient Pole  port_option=ee.enum.threePhasePort.composite  SRated=5e6 A*V  VRated=6600 V  FRated=50 Hz  nPolePairs=4  param_option=ee.enum.sm.parameterization.standard  fieldCircuitParameterization_option=ee.enum.sm.fieldparameterization.current  baseEfd=216.54 V  baseIfd=50 A  zero_sequence=ee.enum.park.zerosequence.exclude  axes_param=ee.enum.rotorangle.daxis  Ladu=0.9  Laqu=0.55  L0=0.15  Ll=0.15  Ra=0.011  Lfd=0.2571  Rfd=0.0006  L1d=0.2  R1d=0.0354  L1q=0.2567  R1q=0.0428  Xl=0.15  Xd=1.05  Xq=0.7  X0=0.15  Xdd=0.35  Xddd=0.25  Xqdd=0.325  d_option=ee.enum.circuit.open  Td0d=5.25 s  Tdd=1.75 s  Td0dd=0.03 s  Tddd=0.0214 s  q_option=ee.enum.circuit.open  Tq0dd=0.05 s  Tqdd=0.0232 s  saturation_option=ee.enum.saturation.exclude  saturation_ifd=[0.00, 0.48, 0.76, 1.38, 1.79]  saturation_Vag=[0.00, 0.43, 0.59, 0.71, 0.76]  initialization_option=ee.enum.sm.initialization.electrical  source_type=ee.enum.sm.load_flow_source_type.Swing  Vmag0=6600 V  Vang0=0 deg  Pt0=0.5 A*V  Qt0=0 A*V  minimum_pu=0.95  phase_search_range=[-inf, inf] deg  gmin=1e-6 S  connection_option=ee.enum.Connection.wye  num_q_dampers=1  rotor_offset=-pi / 2 rad  pu_psid_specify=on  pu_psid_priority=High  pu_psid=0  pu_psid_nominal_specify=off  pu_psid_nominal_value=1  pu_psid_nominal_unit=1  pu_psiq_specify=on  pu_psiq_priority=High  pu_psiq=0  pu_psiq_nominal_specify=off  pu_psiq_nominal_value=1  pu_psiq_nominal_unit=1  pu_psifd_specify=on  pu_psifd_priority=High  pu_psifd=0  pu_psifd_nominal_specify=off  pu_psifd_nominal_value=1  pu_psifd_nominal_unit=1  pu_psi1d_specify=on  pu_psi1d_priority=High  pu_psi1d=0  pu_psi1d_nominal_specify=off  pu_psi1d_nominal_value=1  pu_psi1d_nominal_unit=1  pu_psi1q_specify=on  pu_psi1q_priority=High  pu_psi1q=0  pu_psi1q_nominal_specify=off  pu_psi1q_nominal_value=1  pu_psi1q_nominal_unit=1  angular_position_diff_specify=on  angular_position_diff_priority=High  angular_position_diff=0 deg  angular_position_diff_nominal_specify=off  angular_position_diff_nominal_value=1  angular_position_diff_nominal_unit=deg  Tmeas=298.15 K  alpha=3.93e-3 1/K  stator_thermal_mass=100 J/K  rotor_thermal_mass=200 J/K  temperatureA_specify=off  temperatureA_priority=High  temperatureA=25 degC  temperatureA_nominal_specify=off  temperatureA_nominal_value=1  temperatureA_nominal_unit=degC  temperatureB_specify=off  temperatureB_priority=High  temperatureB=25 degC  temperatureB_nominal_specify=off  temperatureB_nominal_value=1  temperatureB_nominal_unit=degC  temperatureC_specify=off  temperatureC_priority=High  temperatureC=25 degC  temperatureC_nominal_specify=off  temperatureC_nominal_value=1  temperatureC_nominal_unit=degC  temperatureR_specify=off  temperatureR_priority=High  temperatureR=25 degC  temperatureR_nominal_specify=off  temperatureR_nominal_value=1  temperatureR_nominal_unit=degC
      settings: LogSimulationData=on  InternalSimscapePortConfiguration="{\"Bottom\":[],\"Left\":[{\"id\":\"fd_p\",\"label\":\"fd+\",\"type\":\"foundation.electrical.electrical\"},{\"id\":\"fd_n\",\"label\":\"fd-\",\"type\":\"foundation.electrical.electrical\"},{\"id\":\"R\",\"label\":\"R\",\"type\":\"foundation.mechanical.rotational.rotational\"},{\"id\":\"C\",\"label\":\"C\",\"type\":\"foundation.mechanical.rotational.rotational\"}],\"Right\":[{\"id\":\"pu_output\",\"label\":\"pu\",\"type\":\"output\"},{\"id\":\"N\",\"label\":\"~\",\"type\":\"foundation.electrical.three_phase\"}],\"Top\":[]}"
  Goto12 : Goto  Commented=on  GotoTag=PrefG2  TagVisibility=global
  Goto9 : Goto  Commented=on  GotoTag=CBG2  TagVisibility=global
  Ideal Torque Source : fl_lib/Mechanical/Mechanical Sources/Ideal Torque Source
  Inertia : ee_lib/Electromechanical/Mechanical/Machine Inertia  SRated=5e6 V*A  FRated=50 Hz  nPolePairs=4  inertia_option=2  J=27548 kg*m^2  H=3.525 s*W/V/A  damper_option=2  D=39.0509 N*m/(rad/s)  pu_D=0.01  initialization_option=2  fMechanical0=50 Hz  fElectrical0=50 Hz
      settings: LogSimulationData=on  InternalSimscapePortConfiguration="{\"Bottom\":[],\"Left\":[{\"id\":\"R\",\"label\":\"R\",\"type\":\"foundation.mechanical.rotational.rotational\"}],\"Right\":[],\"Top\":[]}"
  MATLAB Function : MATLAB Function  TreatAsAtomicUnit=on
  MATLAB Function1 : MATLAB Function  TreatAsAtomicUnit=on
  Mechanical Rotational Reference : fl_lib/Mechanical/Rotational Elements/Mechanical Rotational Reference
  Modbus Client Read : modbuslib/Modbus Client Read  Commented=on  RetainClient=No Modbus client available  ClientList=No Modbus client available  ConnectionEndpoint=No Modbus client selected  ServerId=1  RegisterTable={ '1', 'PrefG2', '21', 'Holding Register', 'double', '1'; '2', 'QrefG2', '29', 'Holding Register', 'double', '1'; '3', 'CBG2', '38', 'Coil', 'bit', '1' }  SampleTime=1
  Modbus Client Write : modbuslib/Modbus Client Write  Commented=on  RetainClient=No Modbus client available  ClientList=No Modbus client available  ConnectionEndpoint=No Modbus client selected  ServerId=1  RegisterTable={ '1', 'P_gen2', '1', 'Holding Register', 'double'; '2', 'P_gen2_pu', '5', 'Holding Register', 'double'; '3', 'V_gen2_pu', '9', 'Holding Register', 'double'; '4', 'Q_gen2_pu', '13', 'Holding Register', 'double'; '5', 'freq_gen2_pu', '17', 'Holding Register', 'double'; '6', 'DroopPG2', '25', 'Holding Register', 'double'; '7', 'DroopQG2', '34', 'Holding Register', 'double' }  SampleTime=1
  PS Terminator : fl_lib/Physical Signals/Sinks/PS Terminator
  PS-Simulink Converter : nesl_utility/PS-Simulink Converter  PhysicalDomain=network_engine_domain  SubClassName=ps_output  LeftPortType=input  RightPortType=output  PseudoPeriodic=off  Frequencies=[]  VectorFormat=1-D array  Unit=inherit  AffineConversion=off
  PS-Simulink Converter1 : nesl_utility/PS-Simulink Converter  PhysicalDomain=network_engine_domain  SubClassName=ps_output  LeftPortType=input  RightPortType=output  PseudoPeriodic=off  Frequencies=[]  VectorFormat=1-D array  Unit=inherit  AffineConversion=off
  PS-Simulink Converter2 : nesl_utility/PS-Simulink Converter  PhysicalDomain=network_engine_domain  SubClassName=ps_output  LeftPortType=input  RightPortType=output  PseudoPeriodic=off  Frequencies=[]  VectorFormat=1-D array  Unit=inherit  AffineConversion=off
  Product : Product  Commented=on
  Reactive Power (pu) : ee_lib/Electromechanical/Synchronous/Synchronous Machine Measurement  output_idx=13
      settings: InternalSimscapePortConfiguration="{\"Bottom\":[],\"Left\":[{\"id\":\"pu_input\",\"label\":\"pu\",\"type\":\"input\"}],\"Right\":[{\"id\":\"pu_output\",\"label\":\"o\",\"type\":\"output\"}],\"Top\":[]}"
  Rotor Speed (pu) : ee_lib/Electromechanical/Synchronous/Synchronous Machine Measurement  output_idx=4
      settings: InternalSimscapePortConfiguration="{\"Bottom\":[],\"Left\":[{\"id\":\"pu_input\",\"label\":\"pu\",\"type\":\"input\"}],\"Right\":[{\"id\":\"pu_output\",\"label\":\"o\",\"type\":\"output\"}],\"Top\":[]}"
  Simulink-PS Converter : nesl_utility/Simulink-PS Converter  PhysicalDomain=network_engine_domain  SubClassName=ps_input  LeftPortType=input  RightPortType=output  PseudoPeriodic=off  Frequencies=[]  NoiseDistribution=none  NoiseParameters=[]  Unit=1  AffineConversion=off  FilteringAndDerivatives=provide  SimscapeFilterOrder=1  InputFilterTimeConstant=0.001  UdotUserProvided=0
  Subsystem1 : Subsystem
  Subsystem2 : Subsystem
  Sum{,1..3,6..7} (6 alike) : Sum  Inputs=|+-
  Sum4 : Sum  Inputs=+-
  Sum5 : Sum  Inputs=+-
  Sum8 : Sum
  Sum9 : Sum  Inputs=+-
  Synchronous Machine Field Circuit (pu) : ee_lib/Electromechanical/Synchronous/Synchronous Machine Field Circuit  unit_option=ee.enum.unit.pu  SRated=5e6 V*A  FRated=50 Hz  fieldCircuitParameterization_option=2  baseEfd=92.95 V  baseIfd=50 A  parameterization_option=2  Ladu=1.66  Rfd=0.0006  Xl=0.15  Xd=1.05  Xdd=0.35  Xddd=0.23  d_option=ee.enum.circuit.open  Td0d=5.25 s  Tdd=1.3260 s  Td0dd=0.03 s  Tddd=0.0230 s
      settings: LogSimulationData=on  InternalSimscapePortConfiguration="{\"Bottom\":[],\"Left\":[{\"id\":\"Efd_pu\",\"label\":\"Efd_pu\",\"type\":\"input\"},{\"id\":\"Ifd_pu\",\"label\":\"Ifd_pu\",\"type\":\"output\"}],\"Right\":[{\"id\":\"fd_p\",\"label\":\"fd+\",\"type\":\"foundation.electrical.electrical\"},{\"id\":\"fd_n\",\"label\":\"fd-\",\"type\":\"foundation.electrical.electrical\"}],\"Top\":[]}"
  Terminal Voltage Measurement : ee_lib/Electromechanical/Synchronous/Synchronous Machine Measurement  output_idx=14
      settings: LogSimulationData=on  InternalSimscapePortConfiguration="{\"Bottom\":[],\"Left\":[{\"id\":\"pu_input\",\"label\":\"pu\",\"type\":\"input\"}],\"Right\":[{\"id\":\"pu_output\",\"label\":\"o\",\"type\":\"output\"}],\"Top\":[]}"
  Terminal Voltage PS-Simulink : nesl_utility/PS-Simulink Converter  PhysicalDomain=network_engine_domain  SubClassName=ps_output  LeftPortType=input  RightPortType=output  PseudoPeriodic=off  Frequencies=[]  VectorFormat=1-D array  Unit=1  AffineConversion=off
  Toggle Switch : ToggleSwitchBlock
      settings: Values={{'Off', 'On'}, [0 0.05]}
  Vref : Constant  SampleTime=Ts_AC
  scale by base_torque : fl_lib/Physical Signals/Functions/PS Gain  gain=53051.6 N*m
  Conn1 : PMIOPort  Side=Right
  tag scope: DroopPG2=global, DroopQG2=global, P_gen2=global, P_gen2_pu=global, P_gen_tot=global, Q_gen2_pu=global, V_gen2_pu=global, freq_gen2_pu=global
  wires:
  Gain3/1 -> Sum1/1, Display1/1
  Active Power Reference1/1 -> Gain3/1
  MATLAB Function/1(droopQ2) -> Sum2/2
  [G1QDroop] -> Sum4/2
  Constant1/1 -> Sum4/1
  Sum4/1 -> [DroopQG2], MATLAB Function/2(alpha1), Display/1
  Form / Follow/1(T) -> "E_FD Simulink-PS "/1
  Sum2/1 -> Form / Follow/3(Verror)
  [genMode] -> Form / Follow/1(genMode)
  Sum1/1 -> Form / Follow/2(Qerror)
  [Q_gen2_pu] -> Sum1/2
  Subsystem1/1(in1) -> MATLAB Function/1(in1), [Q_gen2_pu]  "Qgen2"
  Vref/1 -> Sum/1
  Sum/1 -> Sum2/1
  Terminal Voltage PS-Simulink/1 -> [V_gen2_pu], Sum/2  "Vgen2"
  PS-Simulink Converter2/1 -> Subsystem1/1(In1)
  Constant3/1 -> Product/2
  Product/1 -> Modbus Client Write/6
  From12/1 -> Product/1
  From13/1 -> Modbus Client Write/7
  From11/1 -> Modbus Client Write/5
  From10/1 -> Modbus Client Write/4
  From9/1 -> Modbus Client Write/3
  From8/1 -> Modbus Client Write/2
  Modbus Client Read/3 -> Goto9/1
  From7/1 -> Modbus Client Write/1
  Modbus Client Read/2 -> Display4/1
  Sum5/1 -> Sum3/1
  [G1Ref] -> Sum5/2
  Constant2/1 -> Sum5/1
  [G1PDroop] -> [DroopPG2], Display8/1, Sum9/2
  Constant5/1 -> Sum9/1
  Sum9/1 -> MATLAB Function1/2(alpha1), Display7/1
  Subsystem2/1(in) -> MATLAB Function1/1(in1), [P_gen2_pu], Gain4/1
  Form / Follow1/1(T) -> Simulink-PS Converter/1
  Sum7/1 -> Form / Follow1/3(Ferror)
  Sum3/1 -> Form / Follow1/2(Perror)
  [genMode] -> Form / Follow1/1(genMode)
  [P_gen2_pu] -> Sum3/2
  Sum8/1 -> [P_gen_tot]
  [P_gen2] -> Sum8/2
  [P_gen1] -> Sum8/1
  Gain4/1 -> [P_gen2]  "P_2"
  PS-Simulink Converter1/1 -> Subsystem2/1(In1)
  PS-Simulink Converter/1 -> [freq_gen2_pu], Sum6/2  "freq2"
  [freqRef] -> Sum6/1
  Sum6/1 -> Sum7/1
  MATLAB Function1/1(droopP2) -> Sum7/2
  Modbus Client Read/1 -> Goto12/1
  connections:
  Ideal Torque Source/RConn2 -- Mechanical Rotational Reference/LConn1 -- Generator 5MVA1/LConn4
  Inertia/LConn1 -- Generator 5MVA1/LConn3 -- Ideal Torque Source/LConn1
  Conn1/RConn1 -- Generator 5MVA1/RConn2
  Synchronous Machine Field Circuit (pu)/RConn1 -- Generator 5MVA1/LConn1
  Generator 5MVA1/LConn2 -- Synchronous Machine Field Circuit (pu)/RConn2
  PS Terminator/LConn1 -- Synchronous Machine Field Circuit (pu)/LConn2
  "E_FD Simulink-PS "/RConn1 -- Synchronous Machine Field Circuit (pu)/LConn1
  "Active Power (pu) "/LConn1 -- Reactive Power (pu)/LConn1 -- Terminal Voltage Measurement/LConn1 -- Generator 5MVA1/RConn1 -- Rotor Speed (pu)/LConn1
  Terminal Voltage Measurement/RConn1 -- Terminal Voltage PS-Simulink/LConn1
  PS-Simulink Converter2/LConn1 -- Reactive Power (pu)/RConn1
  Simulink-PS Converter/RConn1 -- scale by base_torque/LConn1
  scale by base_torque/RConn1 -- Ideal Torque Source/RConn1
  PS-Simulink Converter/LConn1 -- Rotor Speed (pu)/RConn1
  PS-Simulink Converter1/LConn1 -- "Active Power (pu) "/RConn1

== system Cyber_Physical_Microgrid/Generator and Load Curtailment ==
  Step2 : Step  Time=timeSolarCurtail  SampleTime=Ts_AC
  Step3 : Step  Time=timeACLoadCurtail  SampleTime=Ts_AC
  tag scope: curtailLoad=global, curtailSolar=global
  wires:
  Step3/1 -> [curtailLoad]
  Step2/1 -> [curtailSolar]

== system Cyber_Physical_Microgrid/Grid Forming Following ==
  Grid Forming / Grid Following : MATLAB Function  TreatAsAtomicUnit=on
  Unit Delay2 : UnitDelay  InitialCondition=1  SampleTime=Ts_AC  HasFrameUpgradeWarning=on
  tag scope: genMode=global
  wires:
  Grid Forming / Grid Following/1(genMode) -> Unit Delay2/1
  Unit Delay2/1 -> [genMode]
  [gridEnable] -> Grid Forming / Grid Following/1(gridEnable)
